simulink model "project1"  (R2016a)
settings: Solver=FixedStepAuto  StartTime=0.0  StopTime=2  FixedStep=1e-3  RelTol=1e-3
libraries: fuzblock x1
settings Model: Creator=Lenovo  LastModifiedBy=Lenovo

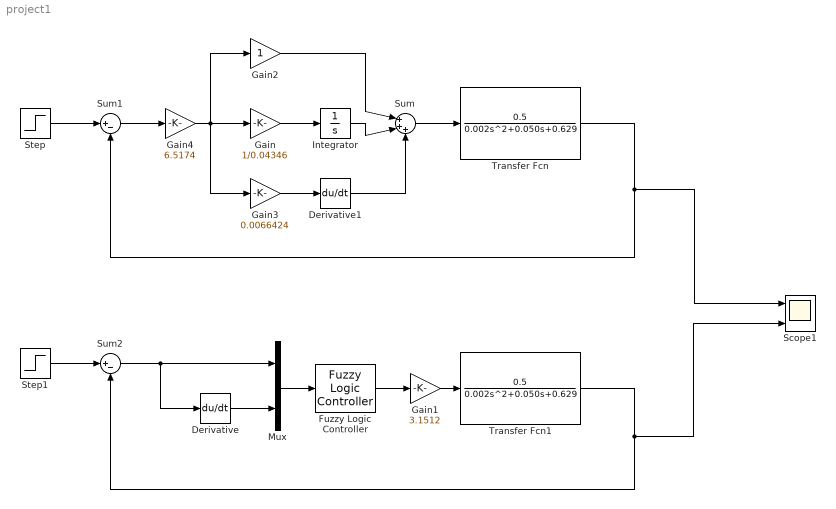
== system project1 ==
  Derivative : Derivative
  Derivative1 : Derivative
  Fuzzy Logic Controller : fuzblock/Fuzzy Logic  Controller  fis='fuzzylogic1'
  Gain : Gain  Gain=1/0.04346
  Gain1 : Gain  Gain=3.1512
  Gain2 : Gain
  Gain3 : Gain  Gain=0.0066424
  Gain4 : Gain  Gain=6.5174
  Integrator : Integrator
  Mux : Mux  Inputs=2
  Scope1 : Scope  NumInputPorts=2
  Step : Step  Time=0  SampleTime=0
  Step1 : Step  Time=0  SampleTime=0
  Sum : Sum  Inputs=|+++
  Sum1 : Sum  Inputs=|+-
  Sum2 : Sum  Inputs=|+-
  Transfer Fcn : TransferFcn  Numerator=[0.5]  Denominator=[0.002 0.050 0.629]
  Transfer Fcn1 : TransferFcn  Numerator=[0.5]  Denominator=[0.002 0.050 0.629]
  wires:
  Step/1 -> Sum1/1
  Transfer Fcn/1 -> Sum1/2, Scope1/1
  Sum/1 -> Transfer Fcn/1
  Derivative/1 -> Mux/2
  Step1/1 -> Sum2/1
  Gain1/1 -> Transfer Fcn1/1
  Mux/1 -> Fuzzy Logic Controller/1
  Fuzzy Logic Controller/1 -> Gain1/1
  Sum2/1 -> Mux/1, Derivative/1
  Derivative1/1 -> Sum/3
  Integrator/1 -> Sum/2
  Gain2/1 -> Sum/1
  Gain/1 -> Integrator/1
  Gain3/1 -> Derivative1/1
  Gain4/1 -> Gain3/1, Gain2/1, Gain/1
  Sum1/1 -> Gain4/1
  Transfer Fcn1/1 -> Sum2/2, Scope1/2
